simulink model "pend_LQR"  (R2018b)
settings: Solver=FixedStepAuto  StartTime=0.0  StopTime=T_final  FixedStep=h  RelTol=1e-3  EnableMultiTasking=on
PreLoadFcn:
  | hwinit
StartFcn:
  | hwinit
values from neighbouring files (symbols this model uses):
  adingain = [1 1]    [data_pend.mat]    (also in hwinit.m = [1, 1]; matlab.mat)
  adinoffs = [-0.2677 -0.1619]    [data_pend.mat]    (also in hwinit.m = [-0.2749;-0.1553]; matlab.mat = [-0.2732 -0.1636])
  amp_out = 0.5    [data_pend.mat]
  angle_bound = [0.287979326579 0 -0.226892802759]    [data_pend.mat]
  angle_real = [-0.0848 -0.0037 0.0549]    [data_pend.mat]
  d_cart = x(1)    [cart_par.m]    (also in data_pend.mat = 4.75430194806; final_est.m = 4.3726; final_estimatien_par.m = X_3(4); matlab.mat = 98.0507473279)
  d_pend = 1.18962575391e-07    [data_pend.mat]    (also in final_est.m = x(1); final_estimatien_par.m = X_3(1); matlab.mat = 1; model.m = X(1))
  daoutgain = 0.9    [data_pend.mat]    (also in hwinit.m = [0.9]; matlab.mat)
  daoutoffs = 0    [data_pend.mat]    (also in hwinit.m = [0]; matlab.mat)
  dsys = c2d(ss(A,B,C,D),h)    [cart_par.m]
  h = 0.01    [calib.m]    (also in data_pend.mat; matlab.mat; model.m; nl_pend_dynamics2.m)
  K = [0.999999843364 1.04891832288]    [data_pend.mat]    (also in matlab.mat = [-0.0462169481806 -7.59777817363 -0.0832109013206 0.00395639; model.m = place(id_pend.A,id_pend.B,eigs); test.mat = [-10908478.8608 -857569.791934 3979815.15158 257262.978008]; testmodel.m = place(id_pend.A,id_pend.B,eigs))
  Km = x(2)    [cart_par.m]    (also in data_pend.mat = 4.080696689; final_est.m = x(3); final_estimatien_par.m = X_3(3); matlab.mat = 82.9763286781)
  l = x(3)    [pend_par2.m]
  mc = x(3)    [cart_par.m]    (also in data_pend.mat = 0.548195745796; final_est.m = 0.5477; final_estimatien_par.m = X_3(5); matlab.mat = 0.49)
  mp = 0.0859999998803    [data_pend.mat]    (also in final_est.m = x(2); final_estimatien_par.m = X_3(2); matlab.mat = 0.085; model.m = 0.085)
  pend = [-0.573 -0.559 -0.487 -0.418 -0.353 -0.29 -0.225 -0.16 -0.094 -0.0247 -0.0037]    [data_pend.mat]    (also in main.m = [-0.573,-0.5590,-0.4870,-0.4180,-0.3530,-0.29,-0.225,-0.16,-; matlab.mat)
  T_final = 10    [data_pend.mat]    (also in main.m = 15; matlab.mat = 30; run_pendulum.m = 15)
  u_out = [0 4.99999999167e-05 0.000199999994667 0.00044999993925 0.000799999658667 0.00124999869792 0.001799996112 0.00244999019593 0.00319997815471 0.0040499557134 0.00499991666708 0.006049852371 ... (1001 elements, 1x1001)]    [data_pend.mat]    (also in main.m = 0.5*sin(5*u_time); matlab.mat = [0 0.002999900003 0.00599920009599 0.00899730072883 0.011993; run_pendulum.m = 0.5*sin(5*u_time))
  u_time = [0 0.01 0.02 0.03 0.04 0.05 0.06 0.07 0.08 0.09 0.1 0.11 ... (1001 elements, 1x1001)]    [data_pend.mat]    (also in main.m = 0:0.01:T_final; matlab.mat = [0 0.01 0.02 0.03 0.04 0.05 0.06 0.07 0.08 0.09 0.1 0.11 ...; run_pendulum.m = 0:0.01:T_final)
  ub_mtr_threshold = 0.16    [data_pend.mat]
  x_init = [0.45556671627 0 0.287807329062 0]    [data_pend.mat]    (also in main.m = [Pos_Pendulum.data(10),0,Angle_Pendulum.data(10),0]; matlab.mat = [0.187021484375 0 -0.0864515625 0]; run_pendulum.m = [Pos_Pendulum.data(10),0,Angle_Pendulum.data(10),0])
undefined symbols (not defined in the file or in its folder): Advantech, DiscIntNeverNeededParam, Discrete, kalman, option, PCI, ref, Time
libraries: sldrtlib x2, ctrlSharedLib x1
settings Model: Creator=zhidayat  LastModifiedBy=dvanhanswijk
settings DataIOCC: LimitDataPoints=on  SaveFormat=Array
settings OptimizationCC: ExpressionDepthLimit=2147483647  LifeSpan=inf
settings DebuggingCC: AllowSymbolicDim=off  StateNameClashWarn=warning  StrictBusMsg=ErrorOnBusTreatedAsVector  SFUnexpectedBacktrackingDiag=warning  SFNoUnconditionalDefaultTransitionDiag=warning  SFExecutionAtInitializationDiag=none
settings HardwareCC: ProdBitPerPointer=32  ProdBitPerSizeT=32  ProdBitPerPtrDiffT=32  ProdLargestAtomicFloat=None  ProdIntDivRoundTo=Undefined  ProdEndianess=Unspecified  ProdWordSize=32  ProdHWDeviceType=32-bit Generic
settings ModelReferenceCC: PropagateSignalLabelsOutOfModel=off
settings SFSimCC: SimUseLocalCustomCode=off
settings RTWCC: RTWUseLocalCustomCode=off
settings CodeAppCC: StateflowObjectComments=on
settings GRTTargetCC: TargetLangStandard=C89/C90 (ANSI)  GeneratePreprocessorConditionals=Disable all  CombineOutputUpdateFcns=off  GRTInterface=on
settings ConfigComp: CovMetricSettings=dw  CovHtmlReporting=on  CovSaveCumulativeToWorkspaceVar=on  CovSaveSingleToWorkspaceVar=on  CovExternalEMLEnable=off

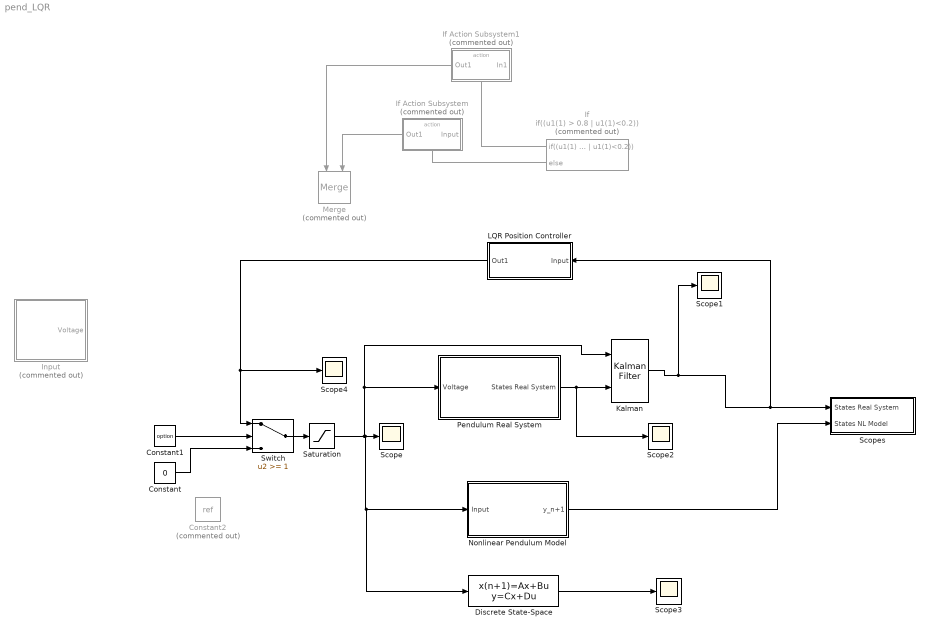
== system pend_LQR ==
  Constant : Constant  Value=0
  Constant1 : Constant  Value=option
  Constant2 : Constant  Commented=on  Value=ref
  Discrete State-Space : DiscreteStateSpace  A=dsys.A  B=dsys.B  C=dsys.C  D=dsys.D  InitialCondition=x_init  SampleTime=h
  If : If  Commented=on  IfExpression=(u1(1) > 0.8 | u1(1)<0.2)
  If Action Subsystem : Subsystem  Commented=on  TreatAsAtomicUnit=on
  If Action Subsystem1 : Subsystem  Commented=on  TreatAsAtomicUnit=on
  "Input " : Subsystem  Commented=on
  "Kalman " : ctrlSharedLib/Kalman Filter  TimeDomain=Discrete-Time  UseCurrentEstimator=on  ModelSource=Individual A, B, C, D matrices  ModelSourceVariable=ss(0.95,1,1,0,1)  A=dsys.A  B=dsys.B  C=dsys.C  D=dsys.D  NumberOfStates=4  NumberOfInputs=1  NumberOfOutputs=2  InitialEstimateSource=Dialog  X0=x_init  P0=10  UseK=off  UseGH=off  NumberOfProcessNoiseInputs=1  G=1  TimeInvariantG=on  H=0  TimeInvariantH=on  Q=kalman.Q  TimeInvariantQ=on  R=kalman.R  TimeInvariantR=on  N=0  TimeInvariantN=on  AddInputPort=on  AddEnablePort=off  OutputEstimatedY=off  OutputP=off  Ts=h
      settings: SourceProductBaseCode=CT
  LQR Position Controller : Subsystem
  Merge : Merge  Commented=on
  Nonlinear Pendulum Model : Subsystem
  "Pendulum Real System " : Subsystem
  Saturation : Saturate  UpperLimit=1  LowerLimit=-1
  Scope{,1..4} (5 alike) : Scope
  "Scopes " : Subsystem
  Switch : Switch  Threshold=1
  wires:
  Nonlinear Pendulum Model/1(y_n+1) -> "Scopes "/2(States NL Model)
  If/2 -> If Action Subsystem/Action
  If/1 -> If Action Subsystem1/Action
  "Kalman "/1 -> Scope1/1, LQR Position Controller/1(Input), "Scopes "/1(States Real System)
  Switch/1 -> Saturation/1
  Constant/1 -> Switch/3
  Constant1/1 -> Switch/2
  "Pendulum Real System "/1(States Real System) -> "Kalman "/2, Scope2/1
  If Action Subsystem/1(Out1) -> Merge/2
  If Action Subsystem1/1(Out1) -> Merge/1
  LQR Position Controller/1(Out1) -> Scope4/1, Switch/1
  Discrete State-Space/1 -> Scope3/1
  Saturation/1 -> Discrete State-Space/1, Nonlinear Pendulum Model/1(Input), Scope/1, "Pendulum Real System "/1(Voltage), "Kalman "/1

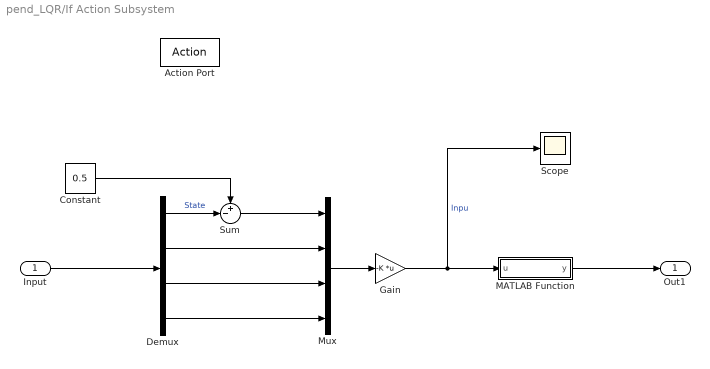
== system pend_LQR/If Action Subsystem ==
  Input : Inport
  Action Port : ActionPort  ActionType=else
  Constant : Constant  Value=0.5
  Demux : Demux
  Gain : Gain  Gain=-K  Multiplication=Matrix(K*u)
  MATLAB Function : MATLAB Function  TreatAsAtomicUnit=on
  Mux : Mux
  Scope : Scope
  Sum : Sum  Inputs=+-|
  Out1 : Outport
  wires:
  Demux/1 -> Sum/2  "State"
  Demux/3 -> Mux/3
  Input/1 -> Demux/1
  Demux/4 -> Mux/4
  Gain/1 -> Scope/1, MATLAB Function/1(u)  "Inpu"
  Mux/1 -> Gain/1
  Sum/1 -> Mux/1
  Demux/2 -> Mux/2
  MATLAB Function/1(y) -> Out1/1
  Constant/1 -> Sum/1

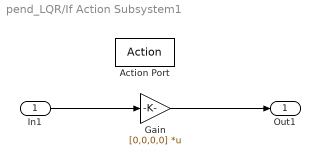
== system pend_LQR/If Action Subsystem1 ==
  In1 : Inport
  Action Port : ActionPort  ActionType=then
  Gain : Gain  Gain=[0,0,0,0]  Multiplication=Matrix(K*u)
  Out1 : Outport
  wires:
  In1/1 -> Gain/1
  Gain/1 -> Out1/1

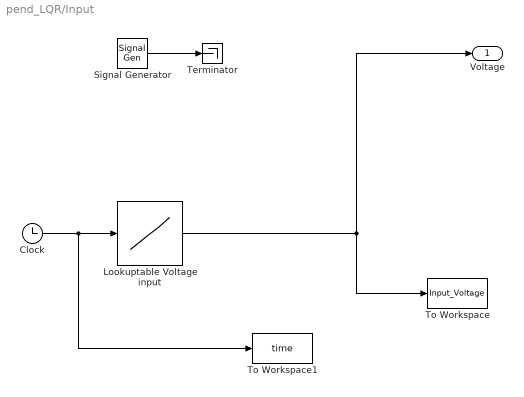
== system pend_LQR/Input  ==
  Clock : Clock
  Lookuptable Voltage input : Lookup_n-D  NumberOfTableDimensions=1  BreakpointsForDimension1=u_time  Table=u_out  InternalRulePriority=Speed  RndMeth=Simplest  InputSameDT=on
  Signal Generator : SignalGenerator  WaveForm=square  Amplitude=amp_out  Frequency=10  Units=rad/sec
  Terminator : Terminator
  To Workspace : ToWorkspace  VariableName=Input_Voltage  SaveFormat=Timeseries  SampleTime=-1
  To Workspace1 : ToWorkspace  VariableName=time  SaveFormat=Timeseries  SampleTime=-1
  Voltage : Outport
  wires:
  Clock/1 -> To Workspace1/1, Lookuptable Voltage input/1
  Lookuptable Voltage input/1 -> Voltage/1, To Workspace/1
  Signal Generator/1 -> Terminator/1

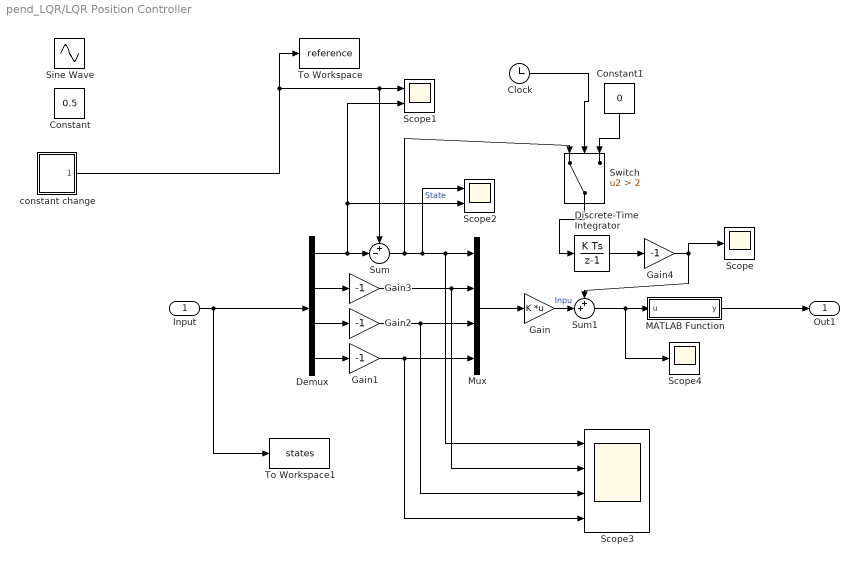
== system pend_LQR/LQR Position Controller ==
  Input : Inport
  Clock : Clock
  Constant : Constant  Value=0.5
  Constant1 : Constant  Value=0
  Demux : Demux
  Discrete-Time Integrator : DiscreteIntegrator  SampleTime=h  ICPrevOutput=DiscIntNeverNeededParam  ICPrevScaledInput=DiscIntNeverNeededParam
  Gain : Gain  Gain=K  Multiplication=Matrix(K*u)
  Gain{1..4} (4 alike) : Gain  Gain=-1
  MATLAB Function : MATLAB Function  TreatAsAtomicUnit=on
  Mux : Mux
  Scope : Scope
  Scope1 : Scope  NumInputPorts=2
  Scope2 : Scope  NumInputPorts=2
  Scope3 : Scope  NumInputPorts=4
  Scope4 : Scope
  Sine Wave : Sin  Amplitude=0.2  Bias=0.5  SampleTime=h
  Sum : Sum  Inputs=+-|
  Sum1 : Sum  Inputs=++|
  Switch : Switch  Criteria=u2 > Threshold  Threshold=2
  To Workspace : ToWorkspace  VariableName=reference  SaveFormat=Timeseries  SampleTime=-1
  To Workspace1 : ToWorkspace  VariableName=states  SaveFormat=Timeseries  SampleTime=-1
  "constant change " : Subsystem
  Out1 : Outport
  wires:
  Input/1 -> To Workspace1/1, Demux/1
  Demux/2 -> Gain3/1
  Mux/1 -> Gain/1
  Demux/1 -> Scope1/2, Scope2/2, Sum/2  "State"
  Demux/3 -> Gain2/1
  Demux/4 -> Gain1/1
  MATLAB Function/1(y) -> Out1/1
  Gain3/1 -> Scope3/2, Mux/2
  Gain2/1 -> Scope3/3, Mux/3
  Gain1/1 -> Scope3/4, Mux/4
  "constant change "/1(Out1) -> To Workspace/1, Sum/1, Scope1/1
  Discrete-Time Integrator/1 -> Gain4/1
  Gain/1 -> Sum1/2  "Inpu"
  Sum1/1 -> Scope4/1, MATLAB Function/1(u)
  Sum/1 -> Switch/1, Scope2/1, Scope3/1, Mux/1
  Clock/1 -> Switch/2
  Constant1/1 -> Switch/3
  Switch/1 -> Discrete-Time Integrator/1
  Gain4/1 -> Sum1/1, Scope/1

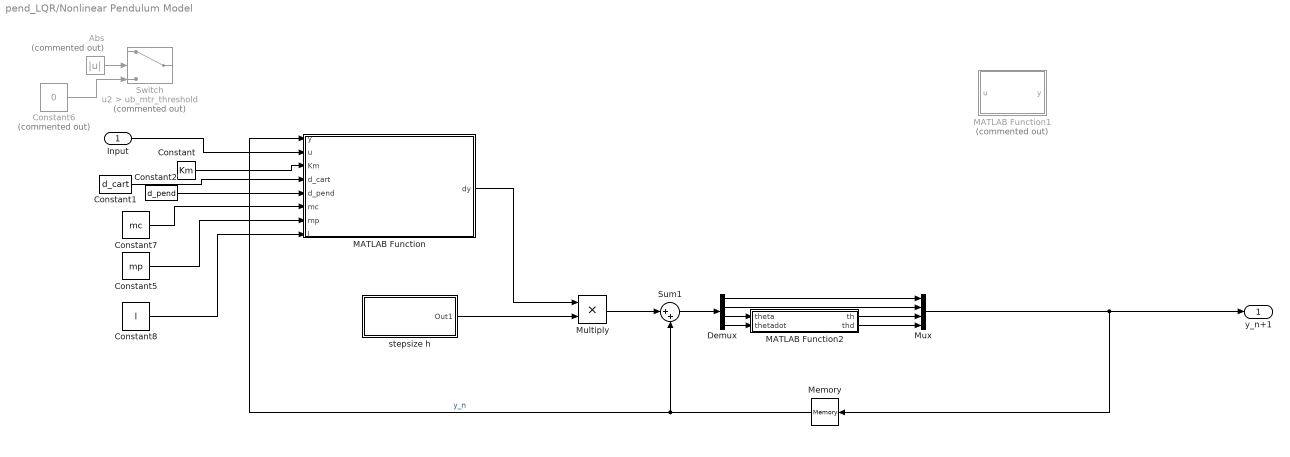
== system pend_LQR/Nonlinear Pendulum Model ==
  Input : Inport
  Abs : Abs  Commented=on
  Constant : Constant  Value=Km
  Constant1 : Constant  Value=d_cart
  Constant2 : Constant  Value=d_pend
  Constant5 : Constant  Value=mp
  Constant6 : Constant  Commented=on  Value=0
  Constant7 : Constant  Value=mc
  Constant8 : Constant  Value=l  SampleTime=h
  Demux : Demux
  MATLAB Function : MATLAB Function  TreatAsAtomicUnit=on
  MATLAB Function1 : MATLAB Function  Commented=on  TreatAsAtomicUnit=on
  MATLAB Function2 : MATLAB Function  TreatAsAtomicUnit=on
  Memory : Memory  InitialCondition=x_init
  Multiply : Product
  Mux : Mux
  Sum1 : Sum  Inputs=|++
  Switch : Switch  Commented=on  Criteria=u2 > Threshold  Threshold=ub_mtr_threshold
  stepsize h : Subsystem
  y_n+1 : Outport
  wires:
  Multiply/1 -> Sum1/1
  Memory/1 -> MATLAB Function/1(y), Sum1/2  "y_n"
  stepsize h/1(Out1) -> Multiply/2
  Constant/1 -> MATLAB Function/3(Km)
  Constant1/1 -> MATLAB Function/4(d_cart)
  Sum1/1 -> Demux/1
  Demux/2 -> Mux/2
  Demux/1 -> Mux/1
  Constant6/1 -> Switch/3
  Input/1 -> MATLAB Function/2(u)
  Abs/1 -> Switch/2
  Constant2/1 -> MATLAB Function/5(d_pend)
  MATLAB Function/1(dy) -> Multiply/1
  Constant5/1 -> MATLAB Function/7(mp)
  Constant7/1 -> MATLAB Function/6(mc)
  Constant8/1 -> MATLAB Function/8(l)
  MATLAB Function2/1(th) -> Mux/3
  Demux/3 -> MATLAB Function2/1(theta)
  Demux/4 -> MATLAB Function2/2(thetadot)
  MATLAB Function2/2(thd) -> Mux/4
  Mux/1 -> Memory/1, y_n+1/1

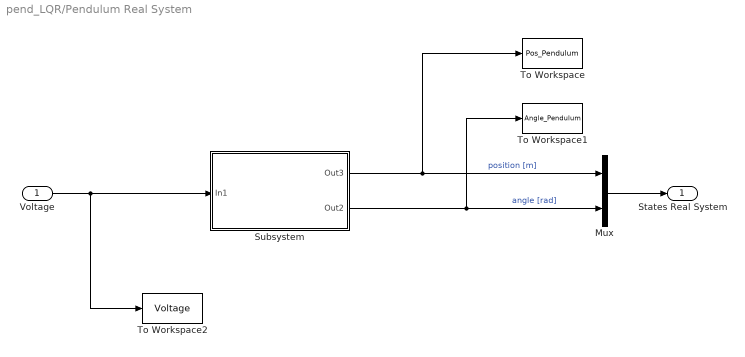
== system pend_LQR/Pendulum Real System  ==
  Voltage : Inport
  Mux : Mux  Inputs=2
  Subsystem : Subsystem  InitFcn=hwinit  StartFcn=hwinit  mask{h=h}
      mask prompts: h "Sample time"
      mask init:
      | hwinit
      mask Display: disp('Pendulum');
  To Workspace : ToWorkspace  VariableName=Pos_Pendulum  SaveFormat=Timeseries  SampleTime=-1
  To Workspace1 : ToWorkspace  VariableName=Angle_Pendulum  SaveFormat=Timeseries  SampleTime=-1
  To Workspace2 : ToWorkspace  VariableName=Voltage  SaveFormat=Timeseries  SampleTime=-1
  States Real System : Outport
  wires:
  Voltage/1 -> To Workspace2/1, Subsystem/1(In1)
  Subsystem/1(Out3) -> To Workspace/1, Mux/1  "position [m]"
  Subsystem/2(Out2) -> Mux/2, To Workspace1/1  "angle [rad]"
  Mux/1 -> States Real System/1

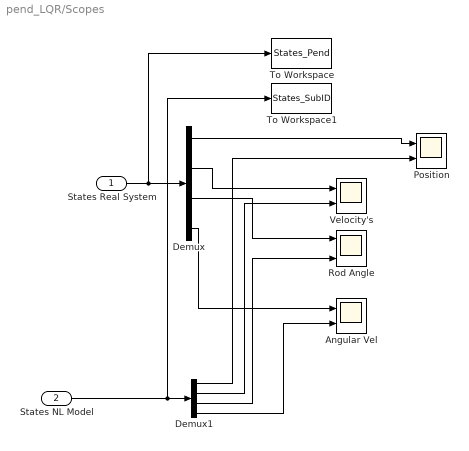
== system pend_LQR/Scopes  ==
  States Real System : Inport
  States NL Model : Inport  Port=2
  "Angular Vel " : Scope  NumInputPorts=2
  Demux : Demux
  Demux1 : Demux
  Position : Scope  NumInputPorts=2
  Rod Angle : Scope  NumInputPorts=2
  To Workspace : ToWorkspace  VariableName=States_Pend  SaveFormat=Timeseries  SampleTime=-1
  To Workspace1 : ToWorkspace  VariableName=States_SubID  SaveFormat=Timeseries  SampleTime=h
  Velocity's : Scope  NumInputPorts=2
  wires:
  States Real System/1 -> To Workspace/1, Demux/1
  Demux/1 -> Position/1
  States NL Model/1 -> To Workspace1/1, Demux1/1
  Demux1/2 -> Velocity's/2
  Demux/2 -> Velocity's/1
  Demux/3 -> Rod Angle/1
  Demux1/3 -> Rod Angle/2
  Demux/4 -> "Angular Vel "/1
  Demux1/4 -> "Angular Vel "/2
  Demux1/1 -> Position/2

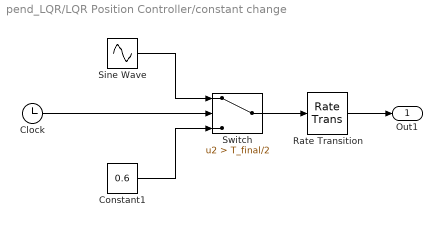
== system pend_LQR/LQR Position Controller/constant change  ==
  Clock : Clock
  Constant1 : Constant  Value=0.6
  Rate Transition : RateTransition  OutPortSampleTime=h
  Sine Wave : Sin  Amplitude=0.2  Bias=0.5  SampleTime=h
  Switch : Switch  Criteria=u2 > Threshold  Threshold=T_final/2
  Out1 : Outport
  wires:
  Sine Wave/1 -> Switch/1
  Constant1/1 -> Switch/3
  Clock/1 -> Switch/2
  Switch/1 -> Rate Transition/1
  Rate Transition/1 -> Out1/1

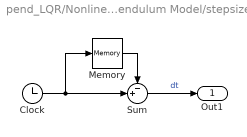
== system pend_LQR/Nonlinear Pendulum Model/stepsize h ==
  Clock : Clock
  Memory : Memory
  Sum : Sum  Inputs=-+|
  Out1 : Outport
  wires:
  Memory/1 -> Sum/1
  Sum/1 -> Out1/1  "dt"
  Clock/1 -> Memory/1, Sum/2

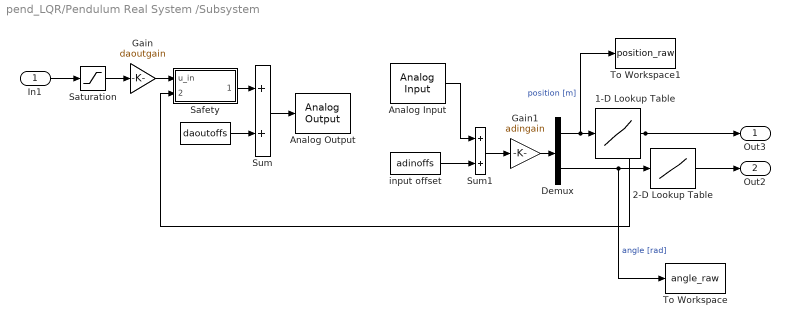
== system pend_LQR/Pendulum Real System /Subsystem ==
  In1 : Inport
  " " : Constant  Value=daoutoffs
  1-D Lookup Table : Lookup_n-D  NumberOfTableDimensions=1  BreakpointsForDimension1=pend  Table=real  InternalRulePriority=Speed  RndMeth=Simplest  InputSameDT=on
  2-D Lookup Table : Lookup_n-D  NumberOfTableDimensions=1  BreakpointsForDimension1=angle_real  BreakpointsForDimension2=[1:3]  Table=angle_bound  InternalRulePriority=Speed  RndMeth=Simplest  InputSameDT=on
  Analog Input : sldrtlib/Analog Input  SampleTime=h  MaxMissedTicks=ticklost  ShowMissedTicks=off  YieldWhenWaiting=on  DrvName=Advantech/PCI-1711  DrvAddress=4294967295  DrvOptions=zeros(1,0)  Channels=adinchannels  RangeMode=2  VoltRange=1  DataType=1
      settings: AttributesFormatString=Advantech\nPCI-1711 [auto]  SourceProductName=Simulink Desktop Real-Time
  Analog Output : sldrtlib/Analog Output  SampleTime=h  MaxMissedTicks=ticklost  ShowMissedTicks=off  YieldWhenWaiting=off  DrvName=Advantech/PCI-1711  DrvAddress=4294967295  DrvOptions=zeros(1,0)  Channels=daoutchannels  RangeMode=2  VoltRange=2  InitialValue=0  FinalValue=0
      settings: AttributesFormatString=Advantech\nPCI-1711 [auto]  SourceProductName=Simulink Desktop Real-Time
  Demux : Demux  Outputs=2
  Gain : Gain  Gain=daoutgain  SaturateOnIntegerOverflow=on  OutDataTypeStr=Inherit: Same as input  ParamDataTypeStr=Inherit: Same as input
  Gain1 : Gain  Gain=adingain  SaturateOnIntegerOverflow=on  OutDataTypeStr=Inherit: Same as input  ParamDataTypeStr=Inherit: Same as input
  Safety : Subsystem
      mask help: The output of the block is restricted to prevent damage to the system. If the cart reaches some safety margins (left: -0.26 and right: 0.26), the output of the block is nullifed. Then the control has to be restarted.
      mask Display: disp('Safety \n margins')
  Saturation : Saturate  UpperLimit=1  LowerLimit=-1
  Sum : Sum  SaturateOnIntegerOverflow=on  OutDataTypeStr=Inherit: Same as first input
  Sum1 : Sum  SaturateOnIntegerOverflow=on  InputSameDT=on  OutDataTypeStr=Inherit: Same as first input
  To Workspace : ToWorkspace  VariableName=angle_raw  SaveFormat=Timeseries  SampleTime=-1
  To Workspace1 : ToWorkspace  VariableName=position_raw  SaveFormat=Timeseries  SampleTime=-1
  input offset : Constant  Value=adinoffs
  Out3 : Outport
  Out2 : Outport  Port=2
  wires:
  Sum1/1 -> Gain1/1
  input offset/1 -> Sum1/2
  Analog Input/1 -> Sum1/1
  Gain1/1 -> Demux/1
  Saturation/1 -> Gain/1
  Sum/1 -> Analog Output/1
  " "/1 -> Sum/2
  In1/1 -> Saturation/1
  Demux/2 -> 2-D Lookup Table/1, To Workspace/1  "angle [rad]"
  Safety/1(u_out) -> Sum/1
  Gain/1 -> Safety/1(u_in)
  Demux/1 -> To Workspace1/1, 1-D Lookup Table/1  "position [m]"
  1-D Lookup Table/1 -> Safety/2(Position), Out3/1
  2-D Lookup Table/1 -> Out2/1

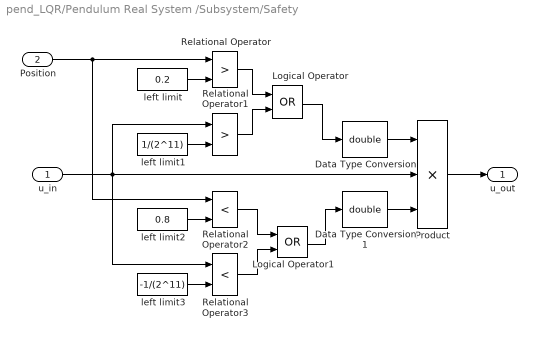
== system pend_LQR/Pendulum Real System /Subsystem/Safety ==
  u_in : Inport
  Position : Inport  Port=2
  Data Type Conversion : DataTypeConversion  OutDataTypeStr=double
  Data Type Conversion1 : DataTypeConversion  OutDataTypeStr=double
  Logical Operator : Logic  Operator=OR  OutDataTypeStr=boolean
  Logical Operator1 : Logic  Operator=OR  OutDataTypeStr=boolean
  Product : Product  Inputs=3  SaturateOnIntegerOverflow=on  InputSameDT=on  OutDataTypeStr=Inherit: Same as first input
  Relational Operator : RelationalOperator  Operator=>  OutDataTypeStr=boolean  RndMeth=Nearest  InputSameDT=on
  Relational Operator1 : RelationalOperator  Operator=>  OutDataTypeStr=boolean  RndMeth=Nearest  InputSameDT=on
  Relational Operator2 : RelationalOperator  Operator=<  OutDataTypeStr=boolean  RndMeth=Nearest  InputSameDT=on
  Relational Operator3 : RelationalOperator  Operator=<  OutDataTypeStr=boolean  RndMeth=Nearest  InputSameDT=on
  left limit : Constant  Value=0.2
  left limit1 : Constant  Value=1/(2^11)
  left limit2 : Constant  Value=0.8
  left limit3 : Constant  Value=-1/(2^11)
  u_out : Outport
  wires:
  left limit1/1 -> Relational Operator1/2
  u_in/1 -> Relational Operator1/1, Relational Operator3/1, Product/2
  Logical Operator1/1 -> Data Type Conversion1/1
  Logical Operator/1 -> Data Type Conversion/1
  left limit/1 -> Relational Operator/2
  Relational Operator/1 -> Logical Operator/1
  Relational Operator1/1 -> Logical Operator/2
  Position/1 -> Relational Operator/1, Relational Operator2/1
  left limit2/1 -> Relational Operator2/2
  Relational Operator2/1 -> Logical Operator1/1
  left limit3/1 -> Relational Operator3/2
  Relational Operator3/1 -> Logical Operator1/2
  Product/1 -> u_out/1
  Data Type Conversion/1 -> Product/1
  Data Type Conversion1/1 -> Product/3

== matlab function pend_LQR/LQR Position Controller/MATLAB Function ==
  data: u input; y output
function y = fcn(u)
ub_mtr_threshold = 0.26;
       y = u + sign(u)*0.9*ub_mtr_threshold;
%        if abs(u) <= ub_mtr_threshold && abs(u) >= lb_mtr_threshold
%            y = sign(u)*(ub_mtr_threshold + 0.02);
%        elseif abs(u) <= lb_mtr_threshold
%            y = 0;
%        else 
%            y = u;
%        end
end

== matlab function pend_LQR/Nonlinear Pendulum Model/MATLAB Function ==
  data: y input; u input; dy output; Km input; d_cart input; d_pend input; mc input; mp input; l input
function dy = nl_pend_dynamics(y,u,Km,d_cart,d_pend,mc,mp,l)
g = 9.81;
dy = zeros(4,1);

dy(1,1) = y(2);
dy(2,1) = 1/((mc+mp)*(1-0.75*mp))*(Km*u - d_cart*y(2) + 3/(2*l)*((l/2)*mp*g*y(3) - d_pend*y(4)) + mp*l*y(4)^2*y(3)/2);
dy(3,1) = y(4);
dy(4,1) = 3/(mp*l^2)*(l*mp*dy(2,1)/2 + l*mp*g*y(3)/2 - d_pend*y(4));

== matlab function pend_LQR/If Action Subsystem/MATLAB Function ==
  data: u input; y output
function y = fcn(u)
ub_mtr_threshold = 0.26;
       y = u + sign(u)*0.9*ub_mtr_threshold;
%        if abs(u) <= ub_mtr_threshold && abs(u) >= lb_mtr_threshold
%            y = sign(u)*(ub_mtr_threshold + 0.02);
%        elseif abs(u) <= lb_mtr_threshold
%            y = 0;
%        else 
%            y = u;
%        end
end

== matlab function pend_LQR/Nonlinear Pendulum Model/MATLAB Function2 ==
  data: theta input; th output; thetadot input; thd output
function [th,thd] = fcn(theta, thetadot)
threshold = 0.26;

if abs(theta) > threshold
    th = threshold*sign(theta);
    thd = 0;
else
    th = theta;
    thd = thetadot;
end

== matlab function pend_LQR/Nonlinear Pendulum Model/MATLAB Function1 ==
  data: u input; y output
function y = fcn(u)
y = u;
if u(1) > 0.8
    y(1) = 0.8;
elseif u(1) < 0.2
    y(1) = 0.2;
    
end
end
